simulink model "F16_model_without_propulsion"  (R2025b)
settings: Solver=VariableStepAuto  StartTime=0.0  StopTime=10.0  RelTol=1e-3
values from neighbouring files (symbols this model uses):
  b = 9.144    [initialization.m]
  c_bar = 3.45    [initialization.m]
  g = 9.81    [initialization.m]
  S = 27.87    [initialization.m]
  xcg = 0.3*c_bar    (= 1.035)    [initialization.m]
  xcgr = 0.35*c_bar    (= 1.2075)    [initialization.m]
undefined symbols (not defined in the file or in its folder): aero_data
libraries: simulink_extras x2
(part 2 of 2)

== system F16_model_without_propulsion/Aerodynamics/Subsystem1/Cn/Aileron Adjustment ==
  alpha : Inport
  beta : Inport  Port=2
  del_lef : Inport  Port=3
  del_a : Inport  Port=4
  Add : Sum
  Cn_del_a_20 : Lookup_n-D  BreakpointsForDimension1=[-20, -15, -10, -5, 0, 5, 10, 15, 20, 25, 30, 35, 40, 45, 50, 55, 60, 70, 80, 90];  BreakpointsForDimension2=[-30, -25, -20, -15, -10, -8, -6, -4, -2, 0, 2, 4, 6, 8, 10, 15, 20, 25, 30];  Table=aero_data.Cn_del_a_20  InternalRulePriority=Speed  RndMeth=Simplest
      settings: InputPortMap=u0,u1
  Cn_del_a_20_lef : Lookup_n-D  BreakpointsForDimension1=[-20, -15, -10, -5, 0, 5, 10, 15, 20, 25, 30, 35, 40, 45];  BreakpointsForDimension2=[-30, -25, -20, -15, -10, -8, -6, -4, -2, 0, 2, 4, 6, 8, 10, 15, 20, 25, 30];  Table=aero_data.Cn_del_a_20_lef  InternalRulePriority=Speed  RndMeth=Simplest
      settings: InputPortMap=u0,u1
  Cn_del_h_0 : Lookup_n-D  BreakpointsForDimension1=[-20, -15, -10, -5, 0, 5, 10, 15, 20, 25, 30, 35, 40, 45, 50, 55, 60, 70, 80, 90];  BreakpointsForDimension2=[-30, -25, -20, -15, -10, -8, -6, -4, -2, 0, 2, 4, 6, 8, 10, 15, 20, 25, 30];  Table=aero_data.Cn_del_h_0  InternalRulePriority=Speed  RndMeth=Simplest
      settings: InputPortMap=u0,u1
  Cn_lef : Lookup_n-D  BreakpointsForDimension1=[-20, -15, -10, -5, 0, 5, 10, 15, 20, 25, 30, 35, 40, 45];  BreakpointsForDimension2=[-30, -25, -20, -15, -10, -8, -6, -4, -2, 0, 2, 4, 6, 8, 10, 15, 20, 25, 30];  Table=aero_data.Cn_lef  InternalRulePriority=Speed  RndMeth=Simplest
      settings: InputPortMap=u0,u1
  Constant : Constant
  Multiply : Gain  Gain=0.04
  Multiply1 : Gain  Gain=0.05
  Product : Product
  Product1 : Product
  Subtract : Sum  Inputs=+--
  Subtract1 : Sum  Inputs=+-
  Subtract2 : Sum  Inputs=+-
  Out1 : Outport
  wires:
  alpha/1 -> Cn_del_a_20_lef/1, Cn_lef/1, Cn_del_h_0/1, Cn_del_a_20/1
  Cn_del_a_20/1 -> Subtract1/1
  beta/1 -> Cn_del_a_20/2, Cn_del_h_0/2, Cn_del_a_20_lef/2, Cn_lef/2
  Cn_del_h_0/1 -> Subtract1/2
  Subtract1/1 -> Add/1, Subtract/3
  Cn_del_a_20_lef/1 -> Subtract/1
  Cn_lef/1 -> Subtract/2
  Subtract/1 -> Product/1
  Constant/1 -> Subtract2/1
  Multiply/1 -> Subtract2/2
  del_lef/1 -> Multiply/1
  Subtract2/1 -> Product/2
  Product/1 -> Add/2
  Add/1 -> Product1/1
  del_a/1 -> Multiply1/1
  Multiply1/1 -> Product1/2
  Product1/1 -> Out1/1

== system F16_model_without_propulsion/Aerodynamics/Subsystem1/Cn/Leading Edge Flap Adjustment ==
  alpha : Inport
  beta : Inport  Port=2
  del_lef : Inport  Port=3
  Cn_del_h_0 : Lookup_n-D  BreakpointsForDimension1=[-20, -15, -10, -5, 0, 5, 10, 15, 20, 25, 30, 35, 40, 45, 50, 55, 60, 70, 80, 90];  BreakpointsForDimension2=[-30, -25, -20, -15, -10, -8, -6, -4, -2, 0, 2, 4, 6, 8, 10, 15, 20, 25, 30];  Table=aero_data.Cn_del_h_0  InternalRulePriority=Speed  RndMeth=Simplest
      settings: InputPortMap=u0,u1
  Cn_lef : Lookup_n-D  BreakpointsForDimension1=[-20, -15, -10, -5, 0, 5, 10, 15, 20, 25, 30, 35, 40, 45];  BreakpointsForDimension2=[-30, -25, -20, -15, -10, -8, -6, -4, -2, 0, 2, 4, 6, 8, 10, 15, 20, 25, 30];  Table=aero_data.Cn_lef  InternalRulePriority=Speed  RndMeth=Simplest
      settings: InputPortMap=u0,u1
  Constant : Constant
  Multiply : Gain  Gain=0.04
  Product : Product
  Subtract : Sum  Inputs=+-
  Subtract1 : Sum  Inputs=+-
  Out1 : Outport
  wires:
  alpha/1 -> Cn_del_h_0/1, Cn_lef/1
  Cn_lef/1 -> Subtract1/1
  Cn_del_h_0/1 -> Subtract1/2
  beta/1 -> Cn_del_h_0/2, Cn_lef/2
  del_lef/1 -> Multiply/1
  Constant/1 -> Subtract/1
  Multiply/1 -> Subtract/2
  Subtract/1 -> Product/2
  Subtract1/1 -> Product/1
  Product/1 -> Out1/1

== system F16_model_without_propulsion/Aerodynamics/Subsystem1/Cn/Roll Rate Damping ==
  alpha : Inport
  del_lef : Inport  Port=2
  p : Inport  Port=3
  Add : Sum
  Cn_p : Lookup_n-D  NumberOfTableDimensions=1  BreakpointsForDimension1=[-20, -15, -10, -5, 0, 5, 10, 15, 20, 25, 30, 35, 40, 45, 50, 55, 60, 70, 80, 90];  Table=aero_data.Cnp  InternalRulePriority=Speed  RndMeth=Simplest
  Constant : Constant
  Constant1 : Constant  Value=25
  Divide : Product  Inputs=*/
  Product : Product
  Product1 : Product
  Subtract : Sum  Inputs=+-
  del_Cn_p_lef : Lookup_n-D  NumberOfTableDimensions=1  BreakpointsForDimension1=[-20, -15, -10, -5, 0, 5, 10, 15, 20, 25, 30, 35, 40, 45];  Table=aero_data.del_Cn_p_lef  InternalRulePriority=Speed  RndMeth=Simplest
  Out1 : Outport
  wires:
  alpha/1 -> del_Cn_p_lef/1, Cn_p/1
  del_Cn_p_lef/1 -> Product/1  "del_Cn_p_lef"
  Cn_p/1 -> Add/1
  del_lef/1 -> Divide/1
  Constant1/1 -> Divide/2
  Constant/1 -> Subtract/1
  Divide/1 -> Subtract/2
  Subtract/1 -> Product/2  "1 - del_lef/25"
  Product/1 -> Add/2
  Add/1 -> Product1/1
  p/1 -> Product1/2
  Product1/1 -> Out1/1

== system F16_model_without_propulsion/Aerodynamics/Subsystem1/Cn/Rudder Adjustment ==
  alpha : Inport
  beta : Inport  Port=2
  del_r : Inport  Port=3
  Cn_del_h_0 : Lookup_n-D  BreakpointsForDimension1=[-20, -15, -10, -5, 0, 5, 10, 15, 20, 25, 30, 35, 40, 45, 50, 55, 60, 70, 80, 90];  BreakpointsForDimension2=[-30, -25, -20, -15, -10, -8, -6, -4, -2, 0, 2, 4, 6, 8, 10, 15, 20, 25, 30];  Table=aero_data.Cn_del_h_0  InternalRulePriority=Speed  RndMeth=Simplest
      settings: InputPortMap=u0,u1
  Cn_del_r_30 : Lookup_n-D  BreakpointsForDimension1=[-20, -15, -10, -5, 0, 5, 10, 15, 20, 25, 30, 35, 40, 45, 50, 55, 60, 70, 80, 90];  BreakpointsForDimension2=[-30, -25, -20, -15, -10, -8, -6, -4, -2, 0, 2, 4, 6, 8, 10, 15, 20, 25, 30];  Table=aero_data.Cn_del_r_30  InternalRulePriority=Speed  RndMeth=Simplest
      settings: InputPortMap=u0,u1
  Multiply : Gain  Gain=1/30
  Product : Product
  Subtract : Sum  Inputs=+-
  Out1 : Outport
  wires:
  beta/1 -> Cn_del_h_0/2, Cn_del_r_30/2
  Cn_del_h_0/1 -> Subtract/2
  Cn_del_r_30/1 -> Subtract/1
  alpha/1 -> Cn_del_h_0/1, Cn_del_r_30/1
  del_r/1 -> Multiply/1
  Subtract/1 -> Product/1
  Multiply/1 -> Product/2
  Product/1 -> Out1/1

== system F16_model_without_propulsion/Aerodynamics/Subsystem1/Cn/Yaw Rate Damping ==
  alpha : Inport
  del_lef : Inport  Port=2
  r : Inport  Port=3
  Add : Sum
  Cn_r : Lookup_n-D  NumberOfTableDimensions=1  BreakpointsForDimension1=[-20, -15, -10, -5, 0, 5, 10, 15, 20, 25, 30, 35, 40, 45, 50, 55, 60, 70, 80, 90];  Table=aero_data.Cnr  InternalRulePriority=Speed  RndMeth=Simplest
  Constant : Constant
  Constant1 : Constant  Value=25
  Divide : Product  Inputs=*/
  Product : Product
  Product1 : Product
  Subtract : Sum  Inputs=+-
  del_Cl_r_lef : Lookup_n-D  NumberOfTableDimensions=1  BreakpointsForDimension1=[-20, -15, -10, -5, 0, 5, 10, 15, 20, 25, 30, 35, 40, 45];  Table=aero_data.del_Cn_r_lef  InternalRulePriority=Speed  RndMeth=Simplest
  Out1 : Outport
  wires:
  Cn_r/1 -> Add/1
  alpha/1 -> del_Cl_r_lef/1, Cn_r/1
  del_Cl_r_lef/1 -> Product/1
  del_lef/1 -> Divide/1
  Divide/1 -> Subtract/2
  Subtract/1 -> Product/2  "1 - del_lef/25"
  Constant/1 -> Subtract/1
  Constant1/1 -> Divide/2
  Product/1 -> Add/2
  Add/1 -> Product1/1
  r/1 -> Product1/2
  Product1/1 -> Out1/1

== system F16_model_without_propulsion/Aerodynamics/Subsystem1/Cx/Leading Edge flap Adjustment ==
  alpha : Inport
  beta : Inport  Port=2
  del_lef : Inport  Port=3
  Constant : Constant
  Constant1 : Constant  Value=25
  Cx_del_h_0 : Lookup_n-D  BreakpointsForDimension1=[-20, -15, -10, -5, 0, 5, 10, 15, 20, 25, 30, 35, 40, 45, 50, 55, 60, 70, 80, 90];  BreakpointsForDimension2=[-30, -25, -20, -15, -10, -8, -6, -4, -2, 0, 2, 4, 6, 8, 10, 15, 20, 25, 30];  Table=aero_data.Cx_del_h_0  InternalRulePriority=Speed  RndMeth=Simplest
      settings: InputPortMap=u0,u1
  Cx_lef : Lookup_n-D  BreakpointsForDimension1=[-20, -15, -10, -5, 0, 5, 10, 15, 20, 25, 30, 35, 40, 45];  BreakpointsForDimension2=[-30, -25, -20, -15, -10, -8, -6, -4, -2, 0, 2, 4, 6, 8, 10, 15, 20, 25, 30];  Table=aero_data.Cx_lef  InternalRulePriority=Speed  RndMeth=Simplest
      settings: InputPortMap=u0,u1
  Divide : Product  Inputs=*/
  Product : Product
  Subtract : Sum  Inputs=+-
  Subtract1 : Sum  Inputs=+-
  Out1 : Outport
  wires:
  alpha/1 -> Cx_lef/1, Cx_del_h_0/1
  Subtract/1 -> Product/1
  Cx_del_h_0/1 -> Subtract/2  "Cx_del_h_10"
  Product/1 -> Out1/1
  Cx_lef/1 -> Subtract/1  "Cx_lef"
  beta/1 -> Cx_lef/2, Cx_del_h_0/2
  del_lef/1 -> Divide/1
  Constant1/1 -> Divide/2
  Constant/1 -> Subtract1/1
  Divide/1 -> Subtract1/2
  Subtract1/1 -> Product/2

== system F16_model_without_propulsion/Aerodynamics/Subsystem1/Cx/Pitching Rate Damping ==
  note: (c_bar*q)/(2*V)
  alpha : Inport
  q : Inport  Port=2
  V : Inport  Port=3
  del_lef : Inport  Port=4
  Add : Sum
  Constant : Constant  Value=c_bar
  Constant1 : Constant  Value=2
  Constant2 : Constant
  Constant3 : Constant  Value=25
  Cxq : Lookup_n-D  NumberOfTableDimensions=1  BreakpointsForDimension1=[-20, -15, -10, -5, 0, 5, 10, 15, 20, 25, 30, 35, 40, 45, 50, 55, 60, 70, 80, 90];  Table=aero_data.Cxq  InternalRulePriority=Speed  RndMeth=Simplest
  Divide : Product  Inputs=*/
  Divide1 : Product  Inputs=*/
  Product{,1..3} (4 alike) : Product
  Subtract1 : Sum  Inputs=+-
  del_Cxq_lef : Lookup_n-D  NumberOfTableDimensions=1  BreakpointsForDimension1=[-20, -15, -10, -5, 0, 5, 10, 15, 20, 25, 30, 35, 40, 45];  Table=aero_data.del_Cxq_lef  InternalRulePriority=Speed  RndMeth=Simplest
  Out1 : Outport
  wires:
  Add/1 -> Product2/1
  Product3/1 -> Add/2
  Cxq/1 -> Add/1  "Cxq"
  del_Cxq_lef/1 -> Product3/1  "del_Cxq_lef"
  Product2/1 -> Out1/1
  alpha/1 -> Cxq/1, del_Cxq_lef/1
  q/1 -> Product/1
  Constant/1 -> Product/2
  Product/1 -> Divide/1
  Constant1/1 -> Product1/1
  V/1 -> Product1/2
  Product1/1 -> Divide/2
  Divide/1 -> Product2/2
  Constant2/1 -> Subtract1/1
  Divide1/1 -> Subtract1/2
  Subtract1/1 -> Product3/2
  del_lef/1 -> Divide1/1
  Constant3/1 -> Divide1/2

== system F16_model_without_propulsion/Aerodynamics/Subsystem1/Cx/Speed Brake ==
  alpha : Inport
  del_sb : Inport  Port=2
  Constant : Constant  Value=60
  Divide : Product  Inputs=*/
  Product : Product
  delCx_sb : Lookup_n-D  NumberOfTableDimensions=1  BreakpointsForDimension1=[-20, -15, -10, -5, 0, 5, 10, 15, 20, 25, 30, 35, 40, 45, 50, 55, 60, 70, 80, 90];  Table=aero_data.del_Cx_sb  InternalRulePriority=Speed  RndMeth=Simplest
  Out1 : Outport
  wires:
  delCx_sb/1 -> Product/1  "del_Cx_sb"
  Product/1 -> Out1/1
  alpha/1 -> delCx_sb/1
  del_sb/1 -> Divide/1
  Constant/1 -> Divide/2
  Divide/1 -> Product/2

== system F16_model_without_propulsion/Aerodynamics/Subsystem1/Cz/Leading Edge Flap Adjustment ==
  alpha : Inport
  beta : Inport  Port=2
  del_lef : Inport  Port=3
  Constant : Constant
  Constant1 : Constant  Value=25
  Cz_del_h_0 : Lookup_n-D  BreakpointsForDimension1=[-20, -15, -10, -5, 0, 5, 10, 15, 20, 25, 30, 35, 40, 45, 50, 55, 60, 70, 80, 90];  BreakpointsForDimension2=[-30, -25, -20, -15, -10, -8, -6, -4, -2, 0, 2, 4, 6, 8, 10, 15, 20, 25, 30];  Table=aero_data.Cz_del_h_0  InternalRulePriority=Speed  RndMeth=Simplest
      settings: InputPortMap=u0,u1
  Cz_lef : Lookup_n-D  BreakpointsForDimension1=[-20, -15, -10, -5, 0, 5, 10, 15, 20, 25, 30, 35, 40, 45];  BreakpointsForDimension2=[-30, -25, -20, -15, -10, -8, -6, -4, -2, 0, 2, 4, 6, 8, 10, 15, 20, 25, 30];  Table=aero_data.Cz_lef  InternalRulePriority=Speed  RndMeth=Simplest
      settings: InputPortMap=u0,u1
  Divide : Product  Inputs=*/
  Product : Product
  Subtract : Sum  Inputs=+-
  Subtract1 : Sum  Inputs=+-
  Out1 : Outport
  wires:
  alpha/1 -> Cz_lef/1, Cz_del_h_0/1
  Subtract/1 -> Product/1
  Cz_del_h_0/1 -> Subtract/2  "Cx_del_h_0"
  Product/1 -> Out1/1
  Cz_lef/1 -> Subtract/1  "Cz_lef"
  beta/1 -> Cz_lef/2, Cz_del_h_0/2
  del_lef/1 -> Divide/1
  Constant1/1 -> Divide/2
  Constant/1 -> Subtract1/1
  Divide/1 -> Subtract1/2
  Subtract1/1 -> Product/2

== system F16_model_without_propulsion/Aerodynamics/Subsystem1/Cz/Pitching Rate Damping ==
  note: (c_bar*q)/(2*V)
  alpha : Inport
  q : Inport  Port=2
  V : Inport  Port=3
  del_lef : Inport  Port=4
  Add : Sum
  Constant : Constant  Value=c_bar
  Constant1 : Constant  Value=2
  Constant2 : Constant
  Constant3 : Constant  Value=25
  Czq : Lookup_n-D  NumberOfTableDimensions=1  BreakpointsForDimension1=[-20, -15, -10, -5, 0, 5, 10, 15, 20, 25, 30, 35, 40, 45, 50, 55, 60, 70, 80, 90];  Table=aero_data.Czq  InternalRulePriority=Speed  RndMeth=Simplest
  Divide : Product  Inputs=*/
  Divide1 : Product  Inputs=*/
  Product{,1..3} (4 alike) : Product
  Subtract1 : Sum  Inputs=+-
  delCzq_lef : Lookup_n-D  NumberOfTableDimensions=1  BreakpointsForDimension1=[-20, -15, -10, -5, 0, 5, 10, 15, 20, 25, 30, 35, 40, 45];  Table=aero_data.delCzq_lef  InternalRulePriority=Speed  RndMeth=Simplest
  Out1 : Outport
  wires:
  Add/1 -> Product2/1
  Product3/1 -> Add/2
  Czq/1 -> Add/1  "Czq"
  delCzq_lef/1 -> Product3/1  "delCzq_lef"
  Product2/1 -> Out1/1
  alpha/1 -> Czq/1, delCzq_lef/1
  q/1 -> Product/1
  Constant/1 -> Product/2
  Product/1 -> Divide/1
  Constant1/1 -> Product1/1
  V/1 -> Product1/2
  Product1/1 -> Divide/2
  Divide/1 -> Product2/2
  Constant2/1 -> Subtract1/1
  Divide1/1 -> Subtract1/2
  Subtract1/1 -> Product3/2
  del_lef/1 -> Divide1/1
  Constant3/1 -> Divide1/2

== system F16_model_without_propulsion/Aerodynamics/Subsystem1/Cz/Speed Brake ==
  alpha : Inport
  del_sb : Inport  Port=2
  Constant : Constant  Value=60
  Divide : Product  Inputs=*/
  Product : Product
  delCz_sb : Lookup_n-D  NumberOfTableDimensions=1  BreakpointsForDimension1=[-20, -15, -10, -5, 0, 5, 10, 15, 20, 25, 30, 35, 40, 45, 50, 55, 60, 70, 80, 90];  Table=aero_data.delCz_sb  InternalRulePriority=Speed  RndMeth=Simplest
  Out1 : Outport
  wires:
  delCz_sb/1 -> Product/1  "delCz_sb"
  Product/1 -> Out1/1
  alpha/1 -> delCz_sb/1
  del_sb/1 -> Divide/1
  Constant/1 -> Divide/2
  Divide/1 -> Product/2

== system F16_model_without_propulsion/Aerodynamics/Subsystem1/C_y/Aileron Adjustment/del_Cy_del_a_20*(1-del_lef//25) ==
  alpha : Inport
  beta : Inport  Port=2
  del_lef : Inport  Port=3
  Constant1 : Constant
  Constant2 : Constant  Value=25
  Cy_del_a_20_lef : Lookup_n-D  BreakpointsForDimension1=[-20, -15, -10, -5, 0, 5, 10, 15, 20, 25, 30, 35, 40, 45];  BreakpointsForDimension2=[-30, -25, -20, -15, -10, -8, -6, -4, -2, 0, 2, 4, 6, 8, 10, 15, 20, 25, 30];  Table=aero_data.Cy_del_a_20_lef  InternalRulePriority=Speed  RndMeth=Simplest
      settings: InputPortMap=u0,u1
  Cy_lef : Lookup_n-D  BreakpointsForDimension1=[-20, -15, -10, -5, 0, 5, 10, 15, 20, 25, 30, 35, 40, 45];  BreakpointsForDimension2=[-30, -25, -20, -15, -10, -8, -6, -4, -2, 0, 2, 4, 6, 8, 10, 15, 20, 25, 30];  Table=aero_data.Cy_lef  InternalRulePriority=Speed  RndMeth=Simplest
      settings: InputPortMap=u0,u1
  Divide1 : Product  Inputs=*/
  Product2 : Product
  Subtract2 : Sum  Inputs=+-
  Subtract3 : Sum  Inputs=+-
  Out1 : Outport
  wires:
  Constant1/1 -> Subtract3/1
  alpha/1 -> Cy_lef/1, Cy_del_a_20_lef/1
  beta/1 -> Cy_lef/2, Cy_del_a_20_lef/2
  Subtract3/1 -> Product2/2  "1 - del_lef/25"
  Subtract2/1 -> Product2/1
  Cy_lef/1 -> Subtract2/2  "Cy_lef"
  Constant2/1 -> Divide1/2
  Product2/1 -> Out1/1
  del_lef/1 -> Divide1/1
  Divide1/1 -> Subtract3/2
  Cy_del_a_20_lef/1 -> Subtract2/1  "Cy_del_a_20_lef"

== system F16_model_without_propulsion/Aerodynamics/Subsystem1/C_y/Flap Adjustment/1-del_lef//25 ==
  del_lef1 : Inport
  Constant1 : Constant
  Constant2 : Constant  Value=25
  Divide1 : Product  Inputs=*/
  Subtract3 : Sum  Inputs=+-
  1 - del_lef/25 : Outport
  wires:
  Constant1/1 -> Subtract3/1
  Subtract3/1 -> 1 - del_lef/25/1  "1 - del_lef/25"
  Divide1/1 -> Subtract3/2
  del_lef1/1 -> Divide1/1
  Constant2/1 -> Divide1/2
